simulink model "Experiment_134_cs"  (Simulink 10.1)
settings: Solver=ode8  StartTime=0.0  StopTime=20  FixedStep=1/10  RelTol=1e-3
PreLoadFcn:
  | mbxruntime.callbacks.PreLoadFcn(bdroot);
PostLoadFcn:
  | mbxruntime.callbacks.PostLoadFcn(bdroot);
InitFcn:
  | mbxruntime.callbacks.InitFcn(bdroot);
StartFcn:
  | mbxruntime.callbacks.StartFcn(bdroot);
StopFcn:
  | mbxruntime.callbacks.StopFcn(bdroot);
undefined symbols (not defined in the file or in its folder): acce_1, acce_2, acce_3, brake, steer, steer_1, steer_2, steer_3, t0_1, t0_2, t0_3, throttle, v_1, v_2, v_3, v_4
libraries: simulink x79, simulink_extras x12, PreScanSimulinkLibrary x8
(part 9 of 9)

== system Experiment_134_cs/Ford_Fiesta_Hatchback_2/Dynamics_Simple/Chassis/Bicycle_model_[XYZ]/Y & Yaw_Motion/Configurable Subsystem2 ==
  In1 : Inport
  In2 : Inport  Port=2
  Integrator : Integrator  ExternalReset=level
  Out1 : Outport
  wires:
  In1/1 -> Integrator/1
  In2/1 -> Integrator/2
  Integrator/1 -> Out1/1

== system Experiment_134_cs/Ford_Fiesta_Hatchback_2/Dynamics_Simple/Chassis/Bicycle_model_[XYZ]/Z, Pitch_Motion & Roll_Motion/Configurable Subsystem ==
  In1 : Inport
  Integrator : Integrator  LimitOutput=on  UpperSaturationLimit=5*pi/180  LowerSaturationLimit=-5*pi/180
  Out1 : Outport
  wires:
  In1/1 -> Integrator/1
  Integrator/1 -> Out1/1

== system Experiment_134_cs/Ford_Fiesta_Hatchback_2/Dynamics_Simple/Chassis/Bicycle_model_[XYZ]/Z, Pitch_Motion & Roll_Motion/Configurable Subsystem1 ==
  In1 : Inport
  Integrator : Integrator
  Out1 : Outport
  wires:
  In1/1 -> Integrator/1
  Integrator/1 -> Out1/1

== system Experiment_134_cs/Ford_Fiesta_Hatchback_2/Dynamics_Simple/Chassis/Bicycle_model_[XYZ]/Z, Pitch_Motion & Roll_Motion/Configurable Subsystem2 ==
  In1 : Inport
  Integrator : Integrator
  Out1 : Outport
  wires:
  In1/1 -> Integrator/1
  Integrator/1 -> Out1/1

== system Experiment_134_cs/Ford_Fiesta_Hatchback_2/Dynamics_Simple/Chassis/Bicycle_model_[XYZ]/Z, Pitch_Motion & Roll_Motion/Configurable Subsystem3 ==
  In1 : Inport
  Integrator : Integrator
  Out1 : Outport
  wires:
  In1/1 -> Integrator/1
  Integrator/1 -> Out1/1

== system Experiment_134_cs/Ford_Fiesta_Hatchback_2/Dynamics_Simple/Chassis/Bicycle_model_[XYZ]/Z, Pitch_Motion & Roll_Motion/Configurable Subsystem4 ==
  In1 : Inport
  Integrator : Integrator
  Out1 : Outport
  wires:
  In1/1 -> Integrator/1
  Integrator/1 -> Out1/1

== system Experiment_134_cs/Ford_Fiesta_Hatchback_2/Dynamics_Simple/Chassis/Bicycle_model_[XYZ]/Z, Pitch_Motion & Roll_Motion/Configurable Subsystem5 ==
  In1 : Inport
  Integrator : Integrator
  Out1 : Outport
  wires:
  In1/1 -> Integrator/1
  Integrator/1 -> Out1/1

== system Experiment_134_cs/Ford_Fiesta_Hatchback_2/Dynamics_Simple/Chassis/Bicycle_model_[XYZ]/Z, Pitch_Motion & Roll_Motion/Configurable Subsystem9 ==
  In1 : Inport
  Derivative : Derivative
  Out1 : Outport
  wires:
  In1/1 -> Derivative/1
  Derivative/1 -> Out1/1

== system Experiment_134_cs/Ford_Fiesta_Hatchback_2/Dynamics_Simple/Chassis/FrontTyre/AlphaFront/Enabled Subsystem ==
  In : Inport
  Enable : EnablePort  PropagateVarSize=During execution
  AlphaFront : Fcn  Expr=-atan( (u(2)+u(3)*p.a)/u(1) )
  Alpha : Outport  OutputWhenDisabled=reset  InitialOutput=[0]
  wires:
  AlphaFront/1 -> Alpha/1
  In/1 -> AlphaFront/1

== system Experiment_134_cs/Ford_Fiesta_Hatchback_2/Dynamics_Simple/Chassis/RearTyre/AlphaRear/Enabled Subsystem ==
  In : Inport
  Enable : EnablePort  PropagateVarSize=During execution
  AlphaRear : Fcn  Expr=-atan( (u(2)-u(3)*p.b)/u(1) )
  Alpha : Outport  OutputWhenDisabled=reset  InitialOutput=[0]
  wires:
  AlphaRear/1 -> Alpha/1
  In/1 -> AlphaRear/1

== system Experiment_134_cs/Ford_Fiesta_Hatchback_3/Dynamics_Simple/Chassis/Bicycle_model_[XYZ]/X_Motion/Air&RoadResistance ==
  vx_[ms-1] : Inport
  Gain : Gain  Gain=1/p.Rw
  Road & Aerodyn Resistances : Fcn  Expr=p.Rroad + p.Rair*u^2
  Saturation1 : Saturate  UpperLimit=5/15  LowerLimit=-5/15
  Sign : Signum
  "[ms-1] 2 [rads-1]" : Gain  Gain=1/p.Rw  SaturateOnIntegerOverflow=on  OutDataTypeStr=Inherit: Same as input  ParamDataTypeStr=Inherit: Same as input
  signed load1 : Product  InputSameDT=on  SaturateOnIntegerOverflow=on  OutDataTypeStr=Inherit: Same as first input
  Resistance_Force : Outport
  wires:
  signed load1/1 -> Resistance_Force/1  "F_[N]"
  vx_[ms-1]/1 -> Road & Aerodyn Resistances/1, "[ms-1] 2 [rads-1]"/1
  Saturation1/1 -> Sign/1
  "[ms-1] 2 [rads-1]"/1 -> Saturation1/1
  Road & Aerodyn Resistances/1 -> Gain/1  "ResistanceTorque_[Nm]"
  Sign/1 -> signed load1/2  "sign"
  Gain/1 -> signed load1/1  "Resistance Force_[N]"

== system Experiment_134_cs/Ford_Fiesta_Hatchback_3/Dynamics_Simple/Chassis/Bicycle_model_[XYZ]/X_Motion/BrakeSystem ==
  vx_[ms-1] : Inport
  BrakePressure_[bar] : Inport  Port=2
  Gain : Gain  Gain=1/p.Rw
  Saturation : Saturate  UpperLimit=p.PBrakeMax  LowerLimit=0
  Saturation1 : Saturate  UpperLimit=5/15  LowerLimit=-5/15
  Sign : Signum
  "[ms-1] 2 [rads-1]" : Gain  Gain=1/p.Rw  SaturateOnIntegerOverflow=on  OutDataTypeStr=Inherit: Same as input  ParamDataTypeStr=Inherit: Same as input
  braking Q factor : Gain  Gain=p.Qfac  SaturateOnIntegerOverflow=on  OutDataTypeStr=Inherit: Same as input  ParamDataTypeStr=Inherit: Same as input
  signed load1 : Product  InputSameDT=on  SaturateOnIntegerOverflow=on  OutDataTypeStr=Inherit: Same as first input
  BrakeForce : Outport
  BrakeTorqueAbs : Outport  Port=2
  wires:
  braking Q factor/1 -> BrakeTorqueAbs/1, Gain/1
  BrakePressure_[bar]/1 -> Saturation/1
  Saturation/1 -> braking Q factor/1
  vx_[ms-1]/1 -> "[ms-1] 2 [rads-1]"/1
  Saturation1/1 -> Sign/1
  "[ms-1] 2 [rads-1]"/1 -> Saturation1/1
  Sign/1 -> signed load1/2  "sign"
  signed load1/1 -> BrakeForce/1
  Gain/1 -> signed load1/1

== system Experiment_134_cs/Ford_Fiesta_Hatchback_3/Dynamics_Simple/Chassis/Bicycle_model_[XYZ]/X_Motion/Configurable Subsystem ==
  In1 : Inport
  In2 : Inport  Port=2
  In3 : Inport  Port=3
  Integrator : Integrator  ExternalReset=level  InitialConditionSource=external
  Out1 : Outport
  wires:
  In1/1 -> Integrator/1
  In2/1 -> Integrator/2
  In3/1 -> Integrator/3
  Integrator/1 -> Out1/1

== system Experiment_134_cs/Ford_Fiesta_Hatchback_3/Dynamics_Simple/Chassis/Bicycle_model_[XYZ]/X_Motion/Configurable Subsystem1 ==
  In1 : Inport
  Torsional damping : TransferFcn  Denominator=[0.1 1]
  Out1 : Outport
  wires:
  In1/1 -> Torsional damping/1
  Torsional damping/1 -> Out1/1

== system Experiment_134_cs/Ford_Fiesta_Hatchback_3/Dynamics_Simple/Chassis/Bicycle_model_[XYZ]/X_Motion/Max RPM and zero- velocity detection ==
  note: Set to zero after infinite small time-step
  note: Zero velocity detection
  ax : Inport
  Drive Torque : Inport  Port=2
  Brake Torque : Inport  Port=3
  v0 : Inport  Port=4
  vx : Inport  Port=5
  Abs : Abs
  Abs1 : Abs
  Compare To Zero : simulink/Logic and Bit Operations/Compare To Zero  relop=<=  OutDataTypeStr=boolean  ZeroCross=off
  Compare To Zero1 : simulink/Logic and Bit Operations/Compare To Zero  relop=>=  OutDataTypeStr=boolean  ZeroCross=off
  Compare To Zero2 : simulink/Logic and Bit Operations/Compare To Zero  relop=>=  OutDataTypeStr=boolean  ZeroCross=off
  Compare To Zero3 : simulink/Logic and Bit Operations/Compare To Zero  relop=<=  OutDataTypeStr=boolean  ZeroCross=off
  Configurable Subsystem : Subsystem  BlockChoice=Step  mask{ComputationMode=ComputationMode}
      mask prompts: ComputationMode "Compuation mode:"
      mask init:
      | SetComputationMode(gcb,ComputationMode);
      settings: AttributesFormatString=%<BlockChoice>  OpenFcn=BringToFront(gcb);  MemberBlocks=Discrete Step,Step
      settings: TemplateBlock=|
      | PreScanSimulinkLibrary/Configurable Subsystems/Step Function/Configurable
      | Subsystem
  Constant : Constant
  Constant1 : Constant
  Logical Operator : Logic  AllPortsSameDT=off  OutDataTypeStr=boolean
  Logical Operator1 : Logic  AllPortsSameDT=off  OutDataTypeStr=boolean
  Logical Operator2 : Logic  Operator=NOT  AllPortsSameDT=off  OutDataTypeStr=boolean
  Logical Operator3 : Logic  AllPortsSameDT=off  OutDataTypeStr=boolean
  Logical Operator4 : Logic  Operator=OR  AllPortsSameDT=off  OutDataTypeStr=boolean
  Memory : Memory
  Memory1 : Memory
  Memory2 : Memory
  Product : Product  RndMeth=Zero
  Relational Operator : RelationalOperator  Operator=<  OutDataTypeStr=boolean  RndMeth=Nearest
  SR-Memory : Subsystem
  Sum : Sum  Inputs=|-+
  Switch : Switch  Criteria=u2 ~= 0  Threshold=0.5
  ax is 0 : Constant  Value=0
  ax_out : Outport
  vx_reset : Outport  Port=2
  x0 : Outport  Port=3
  wires:
  Logical Operator4/1 -> Logical Operator1/1
  vx/1 -> Compare To Zero/1, Compare To Zero2/1, Memory2/1, Memory/1  "vx"
  Memory2/1 -> Compare To Zero3/1
  Compare To Zero2/1 -> Logical Operator3/1
  Compare To Zero3/1 -> Logical Operator3/2
  Logical Operator3/1 -> Logical Operator4/2  "zero-crossing backward"
  Memory/1 -> Compare To Zero1/1
  Compare To Zero/1 -> Logical Operator/1
  Compare To Zero1/1 -> Logical Operator/2
  Logical Operator/1 -> Logical Operator4/1  "zero-crossing forward"
  Abs/1 -> Relational Operator/1
  Abs1/1 -> Relational Operator/2
  Drive Torque/1 -> Abs/1
  Brake Torque/1 -> Abs1/1
  Relational Operator/1 -> Logical Operator1/2, Logical Operator2/1
  Logical Operator1/1 -> SR-Memory/2(Set)
  Constant/1 -> SR-Memory/1(Signal)
  Logical Operator2/1 -> SR-Memory/3(Reset)
  SR-Memory/1(Out) -> Sum/1, Memory1/1
  Switch/1 -> ax_out/1
  Sum/1 -> Switch/2
  ax is 0/1 -> Switch/3
  Constant1/1 -> Sum/2
  v0/1 -> Product/1
  Product/1 -> x0/1
  Configurable Subsystem/1(Out1) -> Product/2
  ax/1 -> Switch/1  "ax"
  Memory1/1 -> vx_reset/1  "vx"

== system Experiment_134_cs/Ford_Fiesta_Hatchback_3/Dynamics_Simple/Chassis/Bicycle_model_[XYZ]/Y & Yaw_Motion/Configurable Subsystem ==
  In1 : Inport
  In2 : Inport  Port=2
  Integrator : Integrator  ExternalReset=level
  Out1 : Outport
  wires:
  In1/1 -> Integrator/1
  In2/1 -> Integrator/2
  Integrator/1 -> Out1/1

== system Experiment_134_cs/Ford_Fiesta_Hatchback_3/Dynamics_Simple/Chassis/Bicycle_model_[XYZ]/Y & Yaw_Motion/Configurable Subsystem1 ==
  In1 : Inport
  Integrator : Integrator
  Out1 : Outport
  wires:
  In1/1 -> Integrator/1
  Integrator/1 -> Out1/1

== system Experiment_134_cs/Ford_Fiesta_Hatchback_3/Dynamics_Simple/Chassis/Bicycle_model_[XYZ]/Y & Yaw_Motion/Configurable Subsystem2 ==
  In1 : Inport
  In2 : Inport  Port=2
  Integrator : Integrator  ExternalReset=level
  Out1 : Outport
  wires:
  In1/1 -> Integrator/1
  In2/1 -> Integrator/2
  Integrator/1 -> Out1/1

== system Experiment_134_cs/Ford_Fiesta_Hatchback_3/Dynamics_Simple/Chassis/Bicycle_model_[XYZ]/Z, Pitch_Motion & Roll_Motion/Configurable Subsystem ==
  In1 : Inport
  Integrator : Integrator  LimitOutput=on  UpperSaturationLimit=5*pi/180  LowerSaturationLimit=-5*pi/180
  Out1 : Outport
  wires:
  In1/1 -> Integrator/1
  Integrator/1 -> Out1/1

== system Experiment_134_cs/Ford_Fiesta_Hatchback_3/Dynamics_Simple/Chassis/Bicycle_model_[XYZ]/Z, Pitch_Motion & Roll_Motion/Configurable Subsystem1 ==
  In1 : Inport
  Integrator : Integrator
  Out1 : Outport
  wires:
  In1/1 -> Integrator/1
  Integrator/1 -> Out1/1

== system Experiment_134_cs/Ford_Fiesta_Hatchback_3/Dynamics_Simple/Chassis/Bicycle_model_[XYZ]/Z, Pitch_Motion & Roll_Motion/Configurable Subsystem2 ==
  In1 : Inport
  Integrator : Integrator
  Out1 : Outport
  wires:
  In1/1 -> Integrator/1
  Integrator/1 -> Out1/1

== system Experiment_134_cs/Ford_Fiesta_Hatchback_3/Dynamics_Simple/Chassis/Bicycle_model_[XYZ]/Z, Pitch_Motion & Roll_Motion/Configurable Subsystem3 ==
  In1 : Inport
  Integrator : Integrator
  Out1 : Outport
  wires:
  In1/1 -> Integrator/1
  Integrator/1 -> Out1/1

== system Experiment_134_cs/Ford_Fiesta_Hatchback_3/Dynamics_Simple/Chassis/Bicycle_model_[XYZ]/Z, Pitch_Motion & Roll_Motion/Configurable Subsystem4 ==
  In1 : Inport
  Integrator : Integrator
  Out1 : Outport
  wires:
  In1/1 -> Integrator/1
  Integrator/1 -> Out1/1

== system Experiment_134_cs/Ford_Fiesta_Hatchback_3/Dynamics_Simple/Chassis/Bicycle_model_[XYZ]/Z, Pitch_Motion & Roll_Motion/Configurable Subsystem5 ==
  In1 : Inport
  Integrator : Integrator
  Out1 : Outport
  wires:
  In1/1 -> Integrator/1
  Integrator/1 -> Out1/1

== system Experiment_134_cs/Ford_Fiesta_Hatchback_3/Dynamics_Simple/Chassis/Bicycle_model_[XYZ]/Z, Pitch_Motion & Roll_Motion/Configurable Subsystem9 ==
  In1 : Inport
  Derivative : Derivative
  Out1 : Outport
  wires:
  In1/1 -> Derivative/1
  Derivative/1 -> Out1/1

== system Experiment_134_cs/Ford_Fiesta_Hatchback_3/Dynamics_Simple/Chassis/FrontTyre/AlphaFront/Enabled Subsystem ==
  In : Inport
  Enable : EnablePort  PropagateVarSize=During execution
  AlphaFront : Fcn  Expr=-atan( (u(2)+u(3)*p.a)/u(1) )
  Alpha : Outport  OutputWhenDisabled=reset  InitialOutput=[0]
  wires:
  AlphaFront/1 -> Alpha/1
  In/1 -> AlphaFront/1

== system Experiment_134_cs/Ford_Fiesta_Hatchback_3/Dynamics_Simple/Chassis/RearTyre/AlphaRear/Enabled Subsystem ==
  In : Inport
  Enable : EnablePort  PropagateVarSize=During execution
  AlphaRear : Fcn  Expr=-atan( (u(2)-u(3)*p.b)/u(1) )
  Alpha : Outport  OutputWhenDisabled=reset  InitialOutput=[0]
  wires:
  AlphaRear/1 -> Alpha/1
  In/1 -> AlphaRear/1

== system Experiment_134_cs/BMW_Z3_Convertible_1/Dynamics_Simple/Chassis/Bicycle_model_[XYZ]/X_Motion/Max RPM and zero- velocity detection/Configurable Subsystem ==
  Step : Step  Time=0.0001  Before=1  After=0  SampleTime=0
  Out1 : Outport
  wires:
  Step/1 -> Out1/1

== system Experiment_134_cs/BMW_Z3_Convertible_1/Dynamics_Simple/Chassis/Bicycle_model_[XYZ]/X_Motion/Max RPM and zero- velocity detection/SR-Memory ==
  Signal : Inport
  Set : Inport  Port=2
  Reset : Inport  Port=3
  Constant : Constant  Value=0
  Detect Rise Positive : simulink/Logic and Bit Operations/Detect Rise Positive  vinit=0  OutDataTypeStr=uint8
  Detect Rise Positive1 : simulink/Logic and Bit Operations/Detect Rise Positive  vinit=0  OutDataTypeStr=uint8
  Manual Switch : ManualSwitch
  Manual Switch1 : ManualSwitch
  Switch : Switch  Criteria=u2 ~= 0
  Switch1 : Switch  Criteria=u2 ~= 0
  Unit Delay : UnitDelay  SampleTime=-1  HasFrameUpgradeWarning=on
  Out : Outport
  wires:
  Constant/1 -> Switch1/1
  Switch/1 -> Switch1/3
  Switch1/1 -> Unit Delay/1, Out/1
  Manual Switch1/1 -> Switch1/2
  Reset/1 -> Manual Switch1/2, Detect Rise Positive1/1
  Detect Rise Positive1/1 -> Manual Switch1/1
  Signal/1 -> Switch/1
  Unit Delay/1 -> Switch/3
  Set/1 -> Detect Rise Positive/1, Manual Switch/2
  Detect Rise Positive/1 -> Manual Switch/1
  Manual Switch/1 -> Switch/2

== system Experiment_134_cs/Ford_Fiesta_Hatchback_1/Dynamics_Simple/Chassis/Bicycle_model_[XYZ]/X_Motion/Max RPM and zero- velocity detection/Configurable Subsystem ==
  Step : Step  Time=0.0001  Before=1  After=0  SampleTime=0
  Out1 : Outport
  wires:
  Step/1 -> Out1/1

== system Experiment_134_cs/Ford_Fiesta_Hatchback_1/Dynamics_Simple/Chassis/Bicycle_model_[XYZ]/X_Motion/Max RPM and zero- velocity detection/SR-Memory ==
  Signal : Inport
  Set : Inport  Port=2
  Reset : Inport  Port=3
  Constant : Constant  Value=0
  Detect Rise Positive : simulink/Logic and Bit Operations/Detect Rise Positive  vinit=0  OutDataTypeStr=uint8
  Detect Rise Positive1 : simulink/Logic and Bit Operations/Detect Rise Positive  vinit=0  OutDataTypeStr=uint8
  Manual Switch : ManualSwitch
  Manual Switch1 : ManualSwitch
  Switch : Switch  Criteria=u2 ~= 0
  Switch1 : Switch  Criteria=u2 ~= 0
  Unit Delay : UnitDelay  SampleTime=-1  HasFrameUpgradeWarning=on
  Out : Outport
  wires:
  Constant/1 -> Switch1/1
  Switch/1 -> Switch1/3
  Switch1/1 -> Unit Delay/1, Out/1
  Manual Switch1/1 -> Switch1/2
  Reset/1 -> Manual Switch1/2, Detect Rise Positive1/1
  Detect Rise Positive1/1 -> Manual Switch1/1
  Signal/1 -> Switch/1
  Unit Delay/1 -> Switch/3
  Set/1 -> Detect Rise Positive/1, Manual Switch/2
  Detect Rise Positive/1 -> Manual Switch/1
  Manual Switch/1 -> Switch/2

== system Experiment_134_cs/Ford_Fiesta_Hatchback_2/Dynamics_Simple/Chassis/Bicycle_model_[XYZ]/X_Motion/Max RPM and zero- velocity detection/Configurable Subsystem ==
  Step : Step  Time=0.0001  Before=1  After=0  SampleTime=0
  Out1 : Outport
  wires:
  Step/1 -> Out1/1

== system Experiment_134_cs/Ford_Fiesta_Hatchback_2/Dynamics_Simple/Chassis/Bicycle_model_[XYZ]/X_Motion/Max RPM and zero- velocity detection/SR-Memory ==
  Signal : Inport
  Set : Inport  Port=2
  Reset : Inport  Port=3
  Constant : Constant  Value=0
  Detect Rise Positive : simulink/Logic and Bit Operations/Detect Rise Positive  vinit=0  OutDataTypeStr=uint8
  Detect Rise Positive1 : simulink/Logic and Bit Operations/Detect Rise Positive  vinit=0  OutDataTypeStr=uint8
  Manual Switch : ManualSwitch
  Manual Switch1 : ManualSwitch
  Switch : Switch  Criteria=u2 ~= 0
  Switch1 : Switch  Criteria=u2 ~= 0
  Unit Delay : UnitDelay  SampleTime=-1  HasFrameUpgradeWarning=on
  Out : Outport
  wires:
  Constant/1 -> Switch1/1
  Switch/1 -> Switch1/3
  Switch1/1 -> Unit Delay/1, Out/1
  Manual Switch1/1 -> Switch1/2
  Reset/1 -> Manual Switch1/2, Detect Rise Positive1/1
  Detect Rise Positive1/1 -> Manual Switch1/1
  Signal/1 -> Switch/1
  Unit Delay/1 -> Switch/3
  Set/1 -> Detect Rise Positive/1, Manual Switch/2
  Detect Rise Positive/1 -> Manual Switch/1
  Manual Switch/1 -> Switch/2

== system Experiment_134_cs/Ford_Fiesta_Hatchback_3/Dynamics_Simple/Chassis/Bicycle_model_[XYZ]/X_Motion/Max RPM and zero- velocity detection/Configurable Subsystem ==
  Step : Step  Time=0.0001  Before=1  After=0  SampleTime=0
  Out1 : Outport
  wires:
  Step/1 -> Out1/1

== system Experiment_134_cs/Ford_Fiesta_Hatchback_3/Dynamics_Simple/Chassis/Bicycle_model_[XYZ]/X_Motion/Max RPM and zero- velocity detection/SR-Memory ==
  Signal : Inport
  Set : Inport  Port=2
  Reset : Inport  Port=3
  Constant : Constant  Value=0
  Detect Rise Positive : simulink/Logic and Bit Operations/Detect Rise Positive  vinit=0  OutDataTypeStr=uint8
  Detect Rise Positive1 : simulink/Logic and Bit Operations/Detect Rise Positive  vinit=0  OutDataTypeStr=uint8
  Manual Switch : ManualSwitch
  Manual Switch1 : ManualSwitch
  Switch : Switch  Criteria=u2 ~= 0
  Switch1 : Switch  Criteria=u2 ~= 0
  Unit Delay : UnitDelay  SampleTime=-1  HasFrameUpgradeWarning=on
  Out : Outport
  wires:
  Constant/1 -> Switch1/1
  Switch/1 -> Switch1/3
  Switch1/1 -> Unit Delay/1, Out/1
  Manual Switch1/1 -> Switch1/2
  Reset/1 -> Manual Switch1/2, Detect Rise Positive1/1
  Detect Rise Positive1/1 -> Manual Switch1/1
  Signal/1 -> Switch/1
  Unit Delay/1 -> Switch/3
  Set/1 -> Detect Rise Positive/1, Manual Switch/2
  Detect Rise Positive/1 -> Manual Switch/1
  Manual Switch/1 -> Switch/2

== matlab function Ford_Fiesta_Hatchback_2/MATLAB Function ==
  data: u input double; y output double
function y = fcn(u)
u = tand(90-u);
y = u;

== matlab function Ford_Fiesta_Hatchback_3/Velocity_control1/MATLAB Function ==
  data: u input double; tho output double; brk output double
function [tho,brk] = fcn(u)
if u >= 0
    brk = 0;
    tho=u;
else
    tho=0;
    brk =u;
end

== matlab function Ford_Fiesta_Hatchback_3/MATLAB Function ==
  data: u input double; y output double
function y = fcn(u)
u = tand(90-u);
y = u;

== matlab function BMW_Z3_Convertible_1/collision safety rule/collision safety rule ==
  data: d input double; throttle output double; d_min input double; thro input double; bra input double; brake output double
function [throttle,brake] = fcn(d,d_min,thro,bra)
if d<d_min
    throttle = -1;
    brake = 1;
else
    throttle = thro;
    brake = bra;
end

== matlab function Ford_Fiesta_Hatchback_2/Velocity_control1/MATLAB Function ==
  data: u input double; tho output double; brk output double
function [tho,brk] = fcn(u)
if u >= 0
    brk = 0;
    tho=u;
else
    tho=0;
    brk =u;
end

== matlab function BMW_Z3_Convertible_1/collision safety rule/MATLAB Function12 ==
  data: x1 input double; d output double; x2 input double; x3 input double; x4 input double; v1 input double; d_min output double; v2 input double; v3 input double; v4 input double
function [d,d_min] = fcn(x1,x2,x3,x4,v1,v2,v3,v4)
if x1>5.15 && x1<8.62
    if x2>5.15 && x2<8.62
        if (x2-x1)>0
            d = x2-x1;
            v_front = v2;
            t_min = 2*(v1-v_front)/4;
            d_min = (v1-v_front)*t_min;
        else
            if x3>5.15 && x3<8.62
                if (x3-x1)>0
                    d = x3-x1;
                    v_front = v3;
                    t_min = 2*(v1-v_front)/4;
                    d_min = (v1-v_front)*t_min;
                else
                    if x4>5.15 && x4<8.62
                        if (x4-x1)>0
                            d = x4-x1;
                            v_front = v4;
                            t_min = 2*(v1-v_front)/4;
                            d_min = (v1-v_front)*t_min;
                        else
                        end
                    else
                    end
                end
            else
            end
        end
    else
    end
elseif x1>8.62 && x1<11.14
    if x2>8.62 && x2<11.14
        if (x2-x1)>0
            d = x2-x1;
            v_front = v2;
            t_min = 2*(v1-v_front)/4;
            d_min = (v1-v_front)*t_min;
        else
            if x3>8.62 && x3<11.14
                if (x3-x1)>0
                    d = x3-x1;
                    v_front = v3;
                    t_min = 2*(v1-v_front)/4;
                    d_min = (v1-v_front)*t_min;
                else
                    if x4>8.62 && x4<11.14
                        if (x4-x1)>0
                            d = x4-x1;
                            v_front = v4;
                            t_min = 2*(v1-v_front)/4;
                            d_min = (v1-v_front)*t_min;
                        else
                        end
                    else
                    end
                end
            else
            end
        end
    else
    end
end

== matlab function Ford_Fiesta_Hatchback_1/Velocity_control1/MATLAB Function ==
  data: u input double; tho output double; brk output double
function [tho,brk] = fcn(u)
if u >= 0
    brk = 0;
    tho=u;
else
    tho=0;
    brk =u;
end

== matlab function Ford_Fiesta_Hatchback_2/Velocity_control1/MATLAB Function1 ==
  data: u input double; tho output double; brk output double
function [tho,brk] = fcn(u)
if u >= 0
    brk = 0;
    tho=u*100/8.5;
else
    tho=0;
    brk =-7.95*u;
end

== matlab function Ford_Fiesta_Hatchback_3/Velocity_control1/MATLAB Function1 ==
  data: u input double; tho output double; brk output double
function [tho,brk] = fcn(u)
if u >= 0
    brk = 0;
    tho=u*100/8.5;
else
    tho=0;
    brk =-7.95*u;
end

== matlab function Ford_Fiesta_Hatchback_1/MATLAB Function4 ==
  data: time input double; bra output double; brake input double
function bra = fcn(time,brake)
if time <= 0.1
    bra = 0;
else
    bra = brake;
end

== matlab function Ford_Fiesta_Hatchback_1/MATLAB Function1 ==
  data: time input double; thro output double; throttle input double
function thro = fcn(time,throttle)
if time <= 0.1
    thro = 0;
else
    thro = throttle;
end

== matlab function BMW_Z3_Convertible_1/MATLAB Function ==
  data: time input double; bra output double; brake input double
function bra = fcn(time,brake)
if time <= 0.05
    bra = 0;
else
    bra = brake;
end

== matlab function Ford_Fiesta_Hatchback_1/MATLAB Function ==
  data: u input double; y output double
function y = fcn(u)
u = tand(90-u);
y = u;

== matlab function BMW_Z3_Convertible_1/MATLAB Function1 ==
  data: action_2 output double; throttle input double; brake input double; action_3 output double
function [action_2,action_3]= fcn(throttle,brake)
action_2 = throttle*50+50;
action_3 = brake*2.5+2.5;

== matlab function BMW_Z3_Convertible_1/MATLAB Function11 ==
  data: x input double; x1 output double
function x1 = fcn(x)
zhong = 2*(x+2.5)/(150+2.5);
x1 = zhong -1;

== matlab function BMW_Z3_Convertible_1/MATLAB Function2 ==
  data: time input double; thro output double; throttle input double
function thro = fcn(time,throttle)
if time <= 0.05
    thro = 0;
else
    thro = throttle;
end

== matlab function Ford_Fiesta_Hatchback_1/Velocity_control1/MATLAB Function1 ==
  data: u input double; tho output double; brk output double
function [tho,brk] = fcn(u)
if u >= 0
    brk = 0;
    tho=u*100/8.5;
else
    tho=0;
    brk =-7.95*u;
end

== matlab function BMW_Z3_Convertible_1/MATLAB Function3 ==
  data: time input double; x input double; ste output double; steer input double
function ste = fcn(time,x,steer)
if time <= 0.05 || x <= 63
    ste = 0;
else
    ste = steer;
end

== matlab function BMW_Z3_Convertible_1/MATLAB Function10 ==
  data: d_head input double; d_heading output double
function d_heading = fcn(d_head)
zhong = 2*(d_head-0)/(30-0);
d_heading = zhong -1;

== matlab function Ford_Fiesta_Hatchback_2/MATLAB Function6 ==
  data: time input double; thro output double; throttle input double
function thro = fcn(time,throttle)
if time <= 0.1
    thro = 0;
else
    thro = throttle;
end

== matlab function Ford_Fiesta_Hatchback_2/MATLAB Function7 ==
  data: time input double; bra output double; brake input double
function bra = fcn(time,brake)
if time <= 0.1
    bra = 0;
else
    bra = brake;
end

== matlab function BMW_Z3_Convertible_1/offroad safety rule ==
  data: x1 input double; steer output double; y1 input double; ste input double
function steer = fcn(x1,y1,ste)
if x1<84 
    if y1<2.6 
        steer = 1;
    elseif y1>11.14
        steer = -1;
    else
        steer = ste;
    end
elseif x1>94
    if y1<6.12
        steer = 1;
    elseif y1>11.14
        steer = -1;
    else
        steer = ste;
    end
elseif x1>=84 && x1<=94
    if y1>11.14
        steer = -1;
    elseif y1<4.3
        steer = 0.8;
    else
        steer = ste;
    end    
end

== matlab function BMW_Z3_Convertible_1/Reward & Terminal/terminal/terminal_collision/MATLAB Function ==
  data: isdone input double; y output double
function y = fcn(isdone)
if isdone == true
    y=1;
else 
    y=0;
end

== matlab function Ford_Fiesta_Hatchback_3/MATLAB Function6 ==
  data: time input double; thro output double; throttle input double
function thro = fcn(time,throttle)
if time <= 0.1
    thro = 0;
else
    thro = throttle;
end

== matlab function Ford_Fiesta_Hatchback_3/MATLAB Function7 ==
  data: time input double; bra output double; brake input double
function bra = fcn(time,brake)
if time <= 0.1
    bra = 0;
else
    bra = brake;
end

== matlab function BMW_Z3_Convertible_1/MATLAB Function4 ==
  data: d_x1 input double; dx1 output double
function dx1 = fcn(d_x1)
zhong = 2*(d_x1+40)/(40);
dx1 = zhong -1;

== matlab function BMW_Z3_Convertible_1/MATLAB Function5 ==
  data: d_x2 input double; dx2 output double
function dx2 = fcn(d_x2)
zhong = 2*(d_x2+20)/(13+20);
dx2 = zhong -1;

== matlab function BMW_Z3_Convertible_1/MATLAB Function6 ==
  data: d_x3 input double; dx3 output double
function dx3 = fcn(d_x3)
zhong = 2*(d_x3+5)/(25+5);
dx3 = zhong -1;

== matlab function BMW_Z3_Convertible_1/MATLAB Function7 ==
  data: y_1 input double; y1 output double
function y1 = fcn(y_1)
zhong = 2*(y_1-2.75)/(11.35-2.75);
y1 = zhong -1;

== matlab function BMW_Z3_Convertible_1/MATLAB Function8 ==
  data: v1 input double; v output double
function v = fcn(v1)
zhong = 2*(v1-0)/(22-0);
v = zhong -1;

== matlab function BMW_Z3_Convertible_1/MATLAB Function9 ==
  data: a1 input double; a output double
function a = fcn(a1)
zhong = 2*(a1+6)/(6+6);
a = zhong -1;

== matlab function BMW_Z3_Convertible_1/Reward & Terminal/MATLAB Function ==
  data: isdone input double; y output double
function y = fcn(isdone)
if isdone == true
    y=1;
else 
    y=0;
end

== matlab function BMW_Z3_Convertible_1/Reward & Terminal/activate/MATLAB Function ==
  data: d_x_1 input double; r output double; y input double
function r = fcn(d_x_1, y)
if d_x_1 <=7 && d_x_1>=0 && y <= 20.15 && y > 15.8
    r = -abs(20.15 - y)*3;
elseif d_x_1 <0 && d_x_1>=-5 && y <= 20.15 && y >= 18.31
    r = -abs(20.15- y)*2*3;
else
    r = 0;
end

== matlab function BMW_Z3_Convertible_1/Reward & Terminal/activate/MATLAB Function1 ==
  data: d_x_2 input double; r output double; y input double
function r = fcn(d_x_2, y)
if d_x_2 <=7 && d_x_2>=0 && y <= 20.7 && y >= 16.4
    r = -abs(y - 16.4)*2;
elseif d_x_2 <0 && d_x_2>=-5 && y <= 18.31 && y >= 15.8
    r = -abs(y - 16.4)*2*2;
else
    r = 0;
end

== matlab function BMW_Z3_Convertible_1/Reward & Terminal/activate/MATLAB Function2 ==
  data: d_x_3 input double; r output double; y input double
function r = fcn(d_x_3, y)
if d_x_3 <=7 && d_x_3>=0 && y <= 20.7 && y >= 15.8
    r = -abs(20.15 - y)*1;
elseif d_x_3 <0 && d_x_3>=-5 && y <= 20.7 && y >= 18.31
    r = -abs(20.15 - y)*2*1;
else
    r = 0;
end

== matlab function BMW_Z3_Convertible_1/Reward & Terminal/comfortable/MATLAB Function ==
  data: r output double; d_heading input double
function r = fcn(d_heading)
r = -max(d_heading-10, 0);

== matlab function BMW_Z3_Convertible_1/Reward & Terminal/shaping/MATLAB Function ==
  data: r output double; d_x3 input double
function r = fcn(d_x3)
if d_x3 > -5
    r = 100/(d_x3 + 5);
else 
    r = 0;
end

== matlab function BMW_Z3_Convertible_1/Reward & Terminal/terminal/terminal_offroad/MATLAB Function ==
  data: x input double; r output double; y input double; isdone output double
function [r,isdone] = fcn(x,y)
if x>=-2.5 && x<= 82.3
    if y<=2.3 || y>=11.35
        r = -400;
        isdone = 1;
    else 
        r = 0;
        isdone = 0;
    end
elseif x>82.3 && x<= 102.2
    if y>=11.35
        r = -400;
        isdone = 1;
    else 
        r = 0;
        isdone = 0;
    end
elseif x>102.2
    if y<=6.1 || y>=11.35
        r = -400;
        isdone = 1;
    else 
        r = 0;
        isdone = 0;
    end
else
    r = 0;
    isdone = 0;
end

== matlab function BMW_Z3_Convertible_1/Reward & Terminal/terminal/terminal_time_v/MATLAB Function ==
  data: time input double; isdone output double; v input double
function isdone = fcn(time,v)
if time>5
    if v<5
        isdone = 1;
    else 
        isdone = 0;
    end
else 
    isdone = 0;
end

== matlab function BMW_Z3_Convertible_1/Reward & Terminal/terminal/terminal_yaw/MATLAB Function ==
  data: delta_heading input double; r output double; isdone output double
function [r,isdone] = fcn(delta_heading)
if delta_heading > 30
    r = -400;
    isdone = 1;
else 
    r = 0;
    isdone = 0;
end
